simulink model "OptimalMPCInput_mdl"  (Simulink 8.1)
settings: Solver=ode45  StartTime=0.0  StopTime=10.0  RelTol=1e-3
undefined symbols (not defined in the file): F, G, H, K, Nc, Nx, xx
settings Model: Creator=Kostas  LastModifiedBy=Kostas
settings DataIOCC: SignalLoggingSaveFormat=Dataset
settings OptimizationCC: ExpressionDepthLimit=128
settings DebuggingCC: FcnCallInpInsideContextMsg=EnableAllAsError
settings GRTTargetCC: CombineOutputUpdateFcns=on  GRTInterface=off

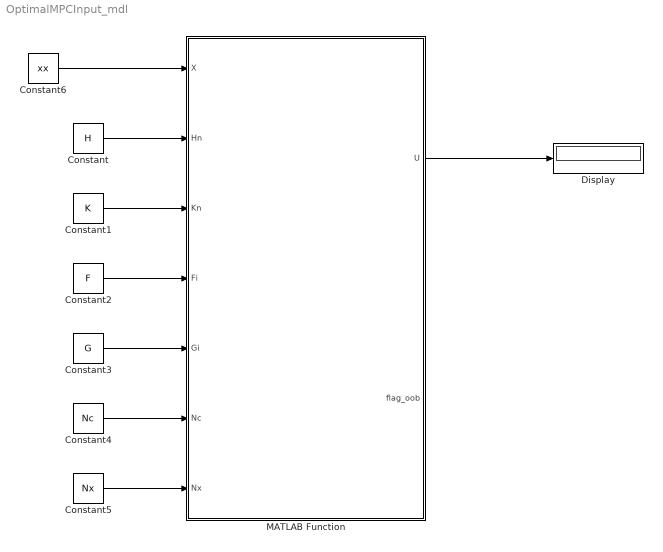
== system OptimalMPCInput_mdl ==
  Constant : Constant  Value=H
  Constant1 : Constant  Value=K
  Constant2 : Constant  Value=F
  Constant3 : Constant  Value=G
  Constant4 : Constant  Value=Nc
  Constant5 : Constant  Value=Nx
  Constant6 : Constant  Value=xx
  Display : Display
  MATLAB Function : MATLAB Function  TreatAsAtomicUnit=on
  wires:
  Constant/1 -> MATLAB Function/2(Hn)
  Constant1/1 -> MATLAB Function/3(Kn)
  Constant2/1 -> MATLAB Function/4(Fi)
  Constant3/1 -> MATLAB Function/5(Gi)
  Constant4/1 -> MATLAB Function/6(Nc)
  Constant5/1 -> MATLAB Function/7(Nx)
  Constant6/1 -> MATLAB Function/1(X)
  MATLAB Function/1(U) -> Display/1

== matlab function MATLAB Function ==
  data: X input double; U output double; Hn input double; Kn input double; Fi input double; Gi input double; Nc input double; Nx input double; flag_oob output double
function[U,flag_oob] = OptimalMPCInput_mdl(X,Hn,Kn,Fi,Gi,Nc,Nx)
%#codegen

tolerance = 1;
nr  = size(Nc,1);
MPT_ABSTOL = 1e-8;
minreg = 0;
X = round(10000*X)/10000;

flag_oob = 0;
%maxSize = max(Nc);

Hi = zeros(1000,Nx);
Ki = zeros(1000,1);

% Find the proper region
abspos = 1;
for ireg = 1:nr
    sumViol = 0;
    isinside = 1;
    

  %  Hi(1:Nc(ireg),1:4) = Hn(abspos:(abspos+Nc(ireg)-1),1:4);
    for i = 1:Nc(ireg)
        for j = 1:Nx
            Hi(i,j) = Hn(abspos + i - 1,j);
        end
    end
    
%    Ki(1:Nc(ireg),1) = Kn(abspos:(abspos+Nc(ireg)-1),1);
    for i = 1:Nc(ireg)
        Ki(i,1) = Kn(abspos + i - 1,1);
    end
    abspos = abspos + Nc(ireg);
    
    F = Fi(ireg,:);
    G = Gi(ireg,:);
    
    nc = Nc(ireg);
    
    for ic = 1:nc
        hx = Hi(ic,:)*X;
        if ((hx - Ki(ic)) > MPT_ABSTOL)
            isinside = 0;
            sumViol = sumViol + (hx - Ki(ic));
        end
    end
    
    if (sumViol < tolerance)
        tolerance = sumViol;
        minreg = ireg;
    end
    % extract the right control law
    if (isinside == 1)
        U = F*X + G;
        return
    end
end
F = Fi(minreg,:);
G = Gi(minreg,:);
U = F*X + G;
flag_oob = 1;
return
